simulink model "tp3partie1"  (Simulink 8.6)
settings: Solver=ode45  StartTime=0.0  StopTime=1000.0  RelTol=1e-3
undefined symbols (not defined in the file): a, am, b, bm, teta10, teta20
settings Model: Creator=AMANI  LastModifiedBy=AMANI
settings DataIOCC: SaveFormat=StructureWithTime
settings OptimizationCC: ExpressionDepthLimit=128
settings DebuggingCC: UnderspecifiedInitializationDetection=Simplified  MergeDetectMultiDrivingBlocksExec=error  SolverPrmCheckMsg=none  FcnCallInpInsideContextMsg=EnableAllAsWarning  StateNameClashWarn=none
settings HardwareCC: ProdIntDivRoundTo=Zero  ProdEndianess=LittleEndian  ProdHWDeviceType=Specified
settings GRTTargetCC: GeneratePreprocessorConditionals=Use local settings
settings ConfigComp: CovModelRefEnable=off

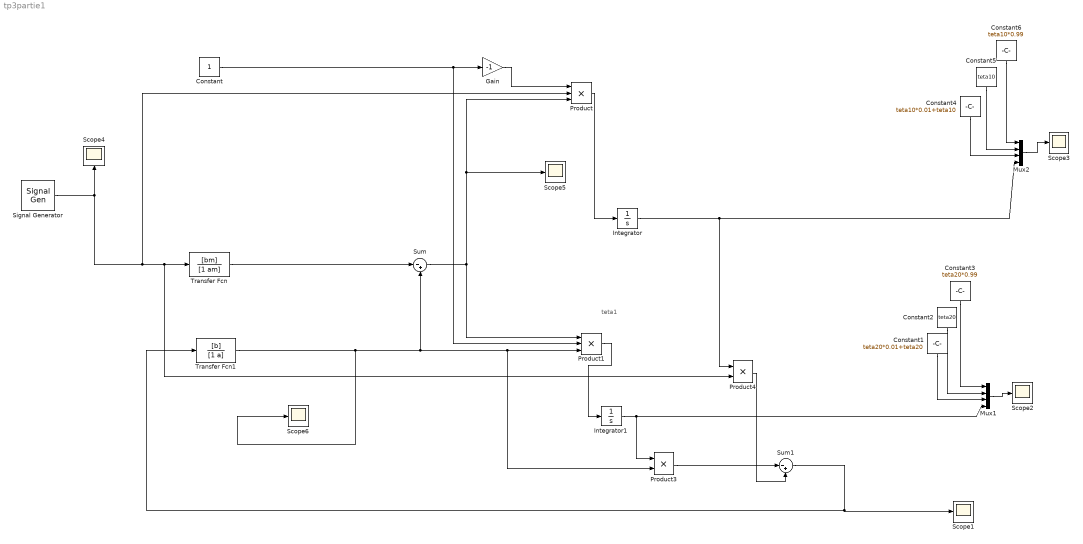
== system tp3partie1 ==
  note: teta1
  Constant : Constant
  Constant1 : Constant  Value=teta20*0.01+teta20
  Constant2 : Constant  Value=teta20
  Constant3 : Constant  Value=teta20*0.99
  Constant4 : Constant  Value=teta10*0.01+teta10
  Constant5 : Constant  Value=teta10
  Constant6 : Constant  Value=teta10*0.99
  Gain : Gain  Gain=-1
  Integrator : Integrator
  Integrator1 : Integrator
  Mux1 : Mux
  Mux2 : Mux
  Product : Product  Inputs=3
  Product1 : Product  Inputs=3
  Product3 : Product
  Product4 : Product
  Scope{1..6} (6 alike) : Scope
  Signal Generator : SignalGenerator  WaveForm=square  Frequency=0.05
  Sum : Sum  Inputs=|-+
  Sum1 : Sum  Inputs=|-+
  Transfer Fcn : TransferFcn  Numerator=[bm]  Denominator=[1 am]
  Transfer Fcn1 : TransferFcn  Numerator=[b]  Denominator=[1 a]
  wires:
  Transfer Fcn1/1 -> Scope6/1, Sum/2, Product3/2, Product1/3
  Transfer Fcn/1 -> Sum/1
  Product/1 -> Integrator/1
  Constant/1 -> Product1/2, Gain/1
  Sum/1 -> Product/3, Scope5/1, Product1/1
  Product1/1 -> Integrator1/1
  Integrator/1 -> Mux2/4, Product4/1
  Product4/1 -> Sum1/2
  Product3/1 -> Sum1/1
  Sum1/1 -> Transfer Fcn1/1, Scope1/1
  Mux1/1 -> Scope2/1
  Constant3/1 -> Mux1/1
  Constant1/1 -> Mux1/3
  Integrator1/1 -> Product3/1, Mux1/4
  Constant2/1 -> Mux1/2
  Mux2/1 -> Scope3/1
  Constant6/1 -> Mux2/1
  Constant4/1 -> Mux2/3
  Constant5/1 -> Mux2/2
  Gain/1 -> Product/1
  Signal Generator/1 -> Scope4/1, Product/2, Product4/2, Transfer Fcn/1
